simulink model "ball_beam_multibody"  (R2022b)
settings: Solver=ode23t  StartTime=0.0  StopTime=stopTime  MaxStep=0.002  RelTol=1e-8  AbsTol=1e-10
model workspace (MAT data in the model file):
  J = 9.99e-06
  Kd = 40
  Kp = 15
  L = 1
  N = 100
  R = 0.015
  d = 0.03
  derivativeOnError = 1
  g = 9.8
  m = 0.111
  reference = 0.25
  stopTime = 10
  thetaMax = inf
undefined symbols (not defined in the file or in its folder): X, Y, Z
libraries: sm_lib x9, nesl_utility x4
settings Model: Creator=shark  LastModifiedBy=shark

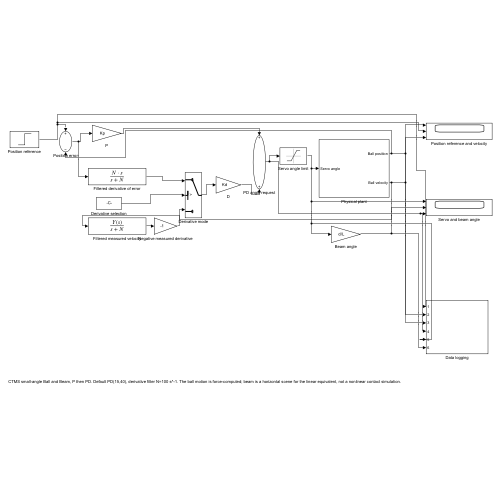
[thumbnail: Simulink's stored preview of the top-level diagram]
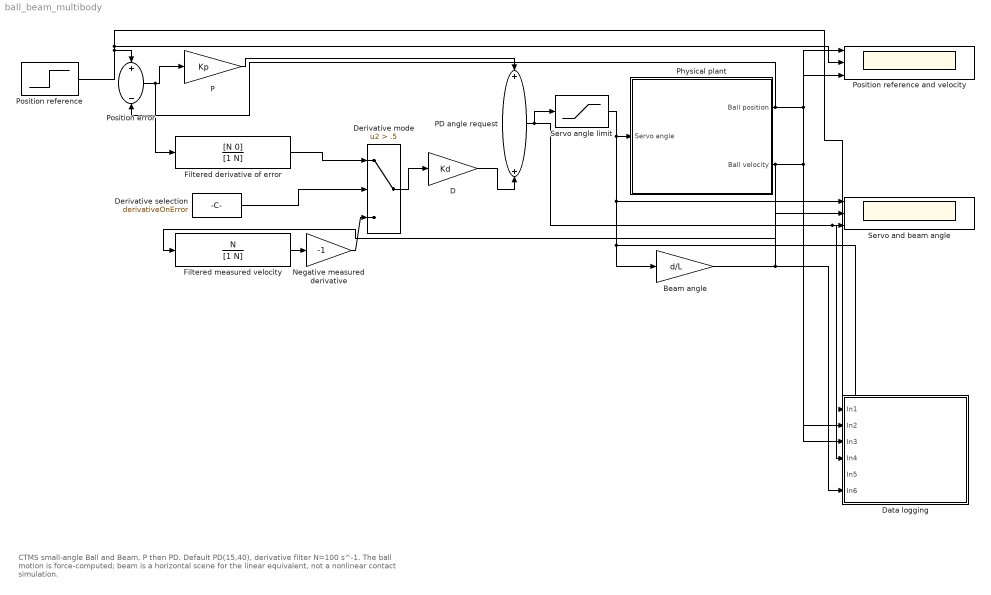
== system ball_beam_multibody ==
  note: CTMS small-angle Ball and Beam, P then PD. Default PD(15,40), derivative filter N=100 s^-1. The ball motion is force-computed; beam is a horizontal scene for the linear equivalent, not a nonlinear contact simulation.
  Beam angle : Gain  Gain=d/L
  D : Gain  Gain=Kd
  Data logging : Subsystem
  Derivative mode : Switch  Criteria=u2 > Threshold  Threshold=.5  SaturateOnIntegerOverflow=off  InputSameDT=off
  Derivative selection : Constant  Value=derivativeOnError
  Filtered derivative of error : TransferFcn  Numerator=[N 0]  Denominator=[1 N]
  Filtered measured velocity : TransferFcn  Numerator=N  Denominator=[1 N]
  Negative measured derivative : Gain  Gain=-1
  P : Gain  Gain=Kp
  PD angle request : Sum
  Physical plant : Subsystem
  Position error : Sum  Inputs=+-
  Position reference : Step  Time=0  After=reference  SampleTime=0
  Position reference and velocity : Scope  NumInputPorts=3
  Servo and beam angle : Scope  NumInputPorts=3
  Servo angle limit : Saturate  UpperLimit=thetaMax  LowerLimit=-thetaMax
  wires:
  Position reference/1 -> Data logging/1(In1), Position reference and velocity/2, Position error/1
  Physical plant/1(Ball position) -> Data logging/2(In2), Position reference and velocity/1, Position error/2
  Position error/1 -> P/1, Filtered derivative of error/1
  Physical plant/2(Ball velocity) -> Data logging/3(In3), Position reference and velocity/3, Filtered measured velocity/1
  Filtered measured velocity/1 -> Negative measured derivative/1
  Filtered derivative of error/1 -> Derivative mode/1
  Derivative selection/1 -> Derivative mode/2
  Negative measured derivative/1 -> Derivative mode/3
  Derivative mode/1 -> D/1
  P/1 -> PD angle request/1
  D/1 -> PD angle request/2
  PD angle request/1 -> Data logging/4(In4), Servo and beam angle/3, Servo angle limit/1
  Servo angle limit/1 -> Beam angle/1, Data logging/5(In5), Servo and beam angle/1, Physical plant/1(Servo angle)
  Beam angle/1 -> Data logging/6(In6), Servo and beam angle/2

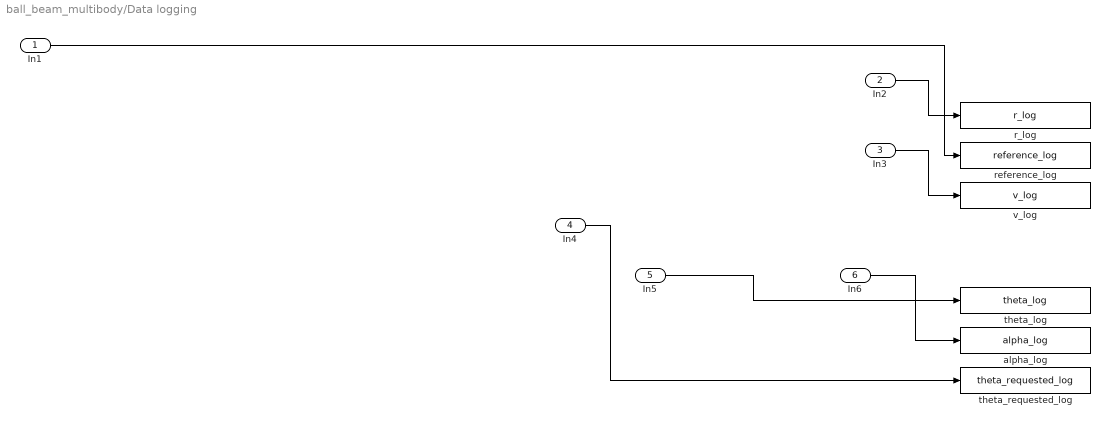
== system ball_beam_multibody/Data logging ==
  In1 : Inport
  In2 : Inport  Port=2
  In3 : Inport  Port=3
  In4 : Inport  Port=4
  In5 : Inport  Port=5
  In6 : Inport  Port=6
  alpha_log : ToWorkspace  VariableName=alpha_log  SaveFormat=Timeseries  SampleTime=-1
  r_log : ToWorkspace  VariableName=r_log  SaveFormat=Timeseries  SampleTime=-1
  reference_log : ToWorkspace  VariableName=reference_log  SaveFormat=Timeseries  SampleTime=-1
  theta_log : ToWorkspace  VariableName=theta_log  SaveFormat=Timeseries  SampleTime=-1
  theta_requested_log : ToWorkspace  VariableName=theta_requested_log  SaveFormat=Timeseries  SampleTime=-1
  v_log : ToWorkspace  VariableName=v_log  SaveFormat=Timeseries  SampleTime=-1
  wires:
  In6/1 -> alpha_log/1
  In5/1 -> theta_log/1
  In4/1 -> theta_requested_log/1
  In1/1 -> reference_log/1
  In3/1 -> v_log/1
  In2/1 -> r_log/1

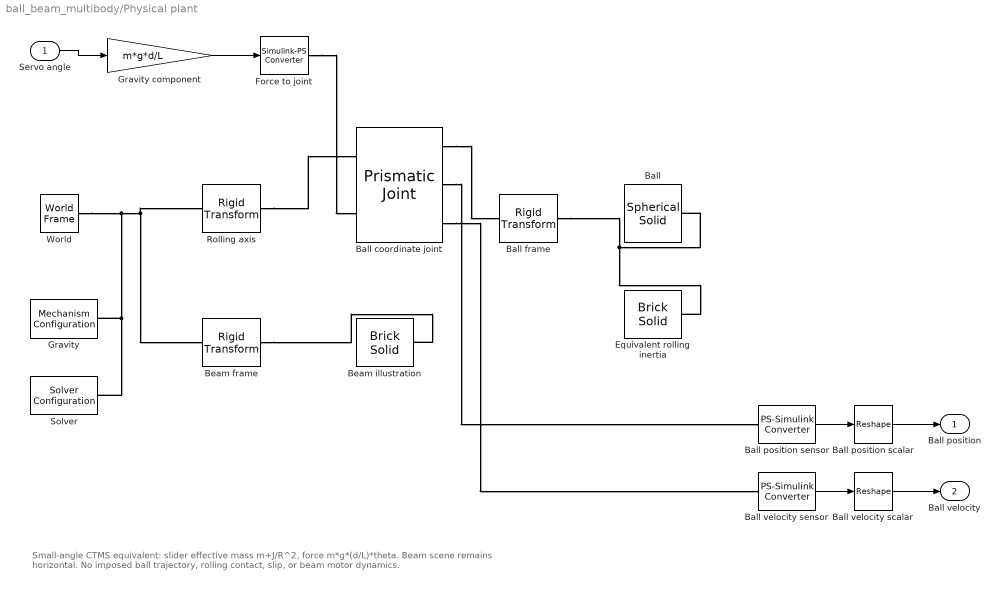
== system ball_beam_multibody/Physical plant ==
  note: Small-angle CTMS equivalent: slider effective mass m+J/R^2, force m*g*(d/L)*theta. Beam scene remains horizontal. No imposed ball trajectory, rolling contact, slip, or beam motor dynamics.
  Servo angle : Inport
  Ball : sm_lib/Body Elements/Spherical Solid  GraphicAmbientColor=[0.15 0.15 0.15 1.0]  BasedOnType=Mass  CenterOfMass=[0 0 0]  CenterOfMassUnits=m  GraphicDiffuseColor=[.85 .25 .12]  Density=1000  DensityUnits=kg/m^3  DoExposeReferenceFrame=on  GraphicEmissiveColor=[0.0 0.0 0.0 1.0]  ExportEntireGeometry=off  SerializedExposedGeometries=<ExposedGeometries/>  SerializedFrames=<Frames/>  MarkerShape=Sphere  MarkerSize=10  GraphicType=FromGeometry  InertiaType=CalculateFromGeometry  Mass=m  MassUnits=kg  MomentsOfInertia=[1 1 1]  MomentsOfInertiaUnits=kg*m^2  GraphicOpacity=1.0  ProductsOfInertia=[0 0 0]  ProductsOfInertiaUnits=kg*m^2  GraphicShininess=75  GraphicSpecularColor=[0.5 0.5 0.5 1.0]  SphereRadius=R  SphereRadiusUnits=m  GraphicVisPropType=SimpleVisualProperties
  Ball coordinate joint : sm_lib/Joints/Prismatic Joint  JointMode=Normal  SenseConstraintForce=off  SenseConstraintForceX=off  SenseConstraintForceY=off  SenseConstraintForceZ=off  SenseConstraintTorque=off  SenseConstraintTorqueX=off  SenseConstraintTorqueY=off  SenseConstraintTorqueZ=off  SenseTotalForce=off  SenseTotalForceX=off  SenseTotalForceY=off  SenseTotalForceZ=off  SenseTotalTorque=off  SenseTotalTorqueX=off  SenseTotalTorqueY=off  SenseTotalTorqueZ=off  CompositeWrenchDir=FollowerOnBase  CompositeWrenchFrame=BaseFrame  EquilibriumPosition=0  EquilibriumPositionUnits=m  SpringStiffness=0  SpringStiffnessUnits=N/m  DampingCoefficient=0  DampingCoefficientUnits=N/(m/s)  TorqueActuationMode=InputTorque  MotionActuationMode=ComputedMotion  SensePosition=on  SenseVelocity=on  SenseAcceleration=off  SenseTorqueForce=off  SenseLowerLimitTorqueForce=off  SenseUpperLimitTorqueForce=off  LowerLimitSpecify=off  LowerLimitBound=-1  LowerLimitBoundUnits=m  LowerLimitStiffness=1e6  LowerLimitStiffnessUnits=N/m  LowerLimitDamping=1e3  LowerLimitDampingUnits=N/(m/s)  LowerLimitTransitionRegionWidth=1e-4  LowerLimitTransitionRegionWidthUnits=m  UpperLimitSpecify=off  UpperLimitBound=1  UpperLimitBoundUnits=m  UpperLimitStiffness=1e6  UpperLimitStiffnessUnits=N/m  UpperLimitDamping=1e3  UpperLimitDampingUnits=N/(m/s)  UpperLimitTransitionRegionWidth=1e-4  UpperLimitTransitionRegionWidthUnits=m  PositionTargetSpecify=on  PositionTargetPriority=High  PositionTargetValue=0  PositionTargetValueUnits=m  VelocityTargetSpecify=on  VelocityTargetPriority=High  VelocityTargetValue=0  VelocityTargetValueUnits=m/s
  Ball frame : sm_lib/Frames and Transforms/Rigid Transform  TranslationMethod=Cartesian  TranslationStandardOffset=0  TranslationLengthUnit=m  TranslationStandardAxis=+Z  TranslationCartesianOffset=[-R 0 0]  TranslationROffset=0  TranslationROffsetUnits=m  TranslationZOffset=0  TranslationZOffsetUnits=m  TranslationThetaOffset=0  TranslationThetaOffsetUnits=deg  RotationMethod=StandardAxis  RotationAngleUnits=deg  RotationStandardAxis=+Y  RotationAngle=-90  RotationArbitraryAxis=[0 0 1]  FollAlignAxisA=+X  BaseAlignAxisA=+Y  FollAlignAxisB=+Y  BaseAlignAxisB=+Z  RotationSequenceAxes=FollowerAxes  RotationSequence=XYX  RotationSequenceAngles=[0 0 0]  RotationSequenceAnglesUnits=deg  RotationMatrix=[1 0 0; 0 1 0; 0 0 1]  Quaternion=[1 0 0 0]
  Ball position scalar : Reshape
  Ball position sensor : nesl_utility/PS-Simulink Converter  PhysicalDomain=network_engine_domain  SubClassName=ps_output  LeftPortType=input  RightPortType=output  PseudoPeriodic=off  Frequencies=[]  VectorFormat=inherit  Unit=m  AffineConversion=off
  Ball velocity scalar : Reshape
  Ball velocity sensor : nesl_utility/PS-Simulink Converter  PhysicalDomain=network_engine_domain  SubClassName=ps_output  LeftPortType=input  RightPortType=output  PseudoPeriodic=off  Frequencies=[]  VectorFormat=inherit  Unit=m/s  AffineConversion=off
  Beam frame : sm_lib/Frames and Transforms/Rigid Transform  TranslationMethod=Cartesian  TranslationStandardOffset=0  TranslationLengthUnit=m  TranslationStandardAxis=+Z  TranslationCartesianOffset=[0 0 -.01]  TranslationROffset=0  TranslationROffsetUnits=m  TranslationZOffset=0  TranslationZOffsetUnits=m  TranslationThetaOffset=0  TranslationThetaOffsetUnits=deg  RotationMethod=StandardAxis  RotationAngleUnits=deg  RotationStandardAxis=+Z  RotationAngle=0  RotationArbitraryAxis=[0 0 1]  FollAlignAxisA=+X  BaseAlignAxisA=+Y  FollAlignAxisB=+Y  BaseAlignAxisB=+Z  RotationSequenceAxes=FollowerAxes  RotationSequence=XYX  RotationSequenceAngles=[0 0 0]  RotationSequenceAnglesUnits=deg  RotationMatrix=[1 0 0; 0 1 0; 0 0 1]  Quaternion=[1 0 0 0]
  Beam illustration : sm_lib/Body Elements/Brick Solid  GraphicAmbientColor=[0.15 0.15 0.15 1.0]  BasedOnType=Mass  BrickDimensions=[L .06 .02]  BrickDimensionUnits=m  CenterOfMass=[0 0 0]  CenterOfMassUnits=m  GraphicDiffuseColor=[0.15 0.4 0.7]  Density=1000  DensityUnits=kg/m^3  DoExposeReferenceFrame=on  GraphicEmissiveColor=[0.0 0.0 0.0 1.0]  ExportEntireGeometry=off  SerializedFrames=<Frames/>  MarkerShape=Sphere  MarkerSize=10  GraphicType=FromGeometry  InertiaType=CalculateFromGeometry  Mass=1  MassUnits=kg  MomentsOfInertia=[1 1 1]  MomentsOfInertiaUnits=kg*m^2  GraphicOpacity=1.0  ProductsOfInertia=[0 0 0]  ProductsOfInertiaUnits=kg*m^2  GraphicShininess=75  GraphicSpecularColor=[0.5 0.5 0.5 1.0]  GraphicVisPropType=SimpleVisualProperties
  Equivalent rolling inertia : sm_lib/Body Elements/Brick Solid  GraphicAmbientColor=[0.15 0.15 0.15 1.0]  BasedOnType=Mass  BrickDimensions=[.01 .01 .01]  BrickDimensionUnits=m  CenterOfMass=[0 0 0]  CenterOfMassUnits=m  GraphicDiffuseColor=[0.5 0.5 0.5]  Density=1000  DensityUnits=kg/m^3  DoExposeReferenceFrame=on  GraphicEmissiveColor=[0.0 0.0 0.0 1.0]  ExportEntireGeometry=off  SerializedFrames=<Frames/>  MarkerShape=Sphere  MarkerSize=10  GraphicType=FromGeometry  InertiaType=CalculateFromGeometry  Mass=J/R^2  MassUnits=kg  MomentsOfInertia=[1 1 1]  MomentsOfInertiaUnits=kg*m^2  GraphicOpacity=0  ProductsOfInertia=[0 0 0]  ProductsOfInertiaUnits=kg*m^2  GraphicShininess=75  GraphicSpecularColor=[0.5 0.5 0.5 1.0]  GraphicVisPropType=SimpleVisualProperties
  Force to joint : nesl_utility/Simulink-PS Converter  PhysicalDomain=network_engine_domain  SubClassName=ps_input  LeftPortType=input  RightPortType=output  PseudoPeriodic=off  Frequencies=[]  NoiseDistribution=none  NoiseParameters=[]  Unit=N  AffineConversion=off  FilteringAndDerivatives=provide  SimscapeFilterOrder=1  InputFilterTimeConstant=0.001  UdotUserProvided=0
  Gravity : sm_lib/Utilities/Mechanism Configuration  UniformGravity=Constant  GravityVector=[0 0 0]  GravityUnits=m/s^2  LinearizationDelta=0.001  JointModeTransitionNonlinearIterations=2
  Gravity component : Gain  Gain=m*g*d/L
  Rolling axis : sm_lib/Frames and Transforms/Rigid Transform  TranslationMethod=Cartesian  TranslationStandardOffset=0  TranslationLengthUnit=m  TranslationStandardAxis=+Z  TranslationCartesianOffset=[0 0 0]  TranslationROffset=0  TranslationROffsetUnits=m  TranslationZOffset=0  TranslationZOffsetUnits=m  TranslationThetaOffset=0  TranslationThetaOffsetUnits=deg  RotationMethod=StandardAxis  RotationAngleUnits=deg  RotationStandardAxis=+Y  RotationAngle=90  RotationArbitraryAxis=[0 0 1]  FollAlignAxisA=+X  BaseAlignAxisA=+Y  FollAlignAxisB=+Y  BaseAlignAxisB=+Z  RotationSequenceAxes=FollowerAxes  RotationSequence=XYX  RotationSequenceAngles=[0 0 0]  RotationSequenceAnglesUnits=deg  RotationMatrix=[1 0 0; 0 1 0; 0 0 1]  Quaternion=[1 0 0 0]
  Solver : nesl_utility/Solver Configuration  PhysicalDomain=network_engine_domain  SubClassName=solver  LeftPortType=input  RightPortType=generic  Tones=[]  Harmonics=[]  SimulateNoise=off  Profile=off  UseLocalSampling=off  EnableSwitchedLinearOptims=on  FrequencyDomain=off  UseCCode=off  RelTol=0.001  AbsTol=0.001  MinStep=1e-09  ToWorkspace=off  RevertToSquareIcSolve=off  NumHomotopyIterations=100  PhasorMode=off  PhasorModeNumHarmonics=1  ConsistencySolver=NEWTON_XTOL_AFTER_FTOL  IndexReductionMethod=DerivativeReplacement  DoDC=off  ResidualTolerance=1e-09  ConsistencyTolSource=GLOBAL  ConsistencyAbsTol=0.001  ConsistencyRelTol=0.001  ConsistencyTolFactor=0.001  UseLocalSolver=off  LocalSolverChoice=NE_BACKWARD_EULER_ADVANCER  ResolveIndetEquations=on  FunctionEvalNumThread=1  LocalSolverSampleTime=0.001  DoFixedCost=off  MaxNonlinIter=3  MaxModeIter=2  ComputeImpulses=off  ImpulseIterations=2  LinearAlgebra=auto  LinearAlgebraNumThread=0  EquationFormulation=NE_TIME_EF  DelaysMemoryBudget=1024  AutomaticFiltering=on  FilteringTimeConstant=0.001  PartitionStorageMethod=AS_NEEDED  PartitionMemoryBudget=1024  PartitionMethod=ROBUST
  World : sm_lib/Frames and Transforms/World Frame
  Ball position : Outport
  Ball velocity : Outport  Port=2
  wires:
  Servo angle/1 -> Gravity component/1
  Gravity component/1 -> Force to joint/1
  Ball position sensor/1 -> Ball position scalar/1
  Ball position scalar/1 -> Ball position/1
  Ball velocity sensor/1 -> Ball velocity scalar/1
  Ball velocity scalar/1 -> Ball velocity/1
  connections:
  Gravity/RConn1 -- World/RConn1 -- Rolling axis/LConn1 -- Beam frame/LConn1 -- Solver/RConn1
  Rolling axis/RConn1 -- Ball coordinate joint/LConn1
  Force to joint/RConn1 -- Ball coordinate joint/LConn2
  Ball coordinate joint/RConn1 -- Ball frame/LConn1
  Ball/RConn1 -- Ball frame/RConn1 -- Equivalent rolling inertia/RConn1
  Beam frame/RConn1 -- Beam illustration/RConn1
  Ball coordinate joint/RConn2 -- Ball position sensor/LConn1
  Ball coordinate joint/RConn3 -- Ball velocity sensor/LConn1
